simulink model "FlatEarth_MATLAB7"  (Simulink 8.1)
settings: Solver=ode45  StartTime=0.0  StopTime=Tstop  RelTol=1e-3
undefined symbols (not defined in the file): constant, deltaApertRAD, deltabhppert, deltaEpertRAD, deltaRpertRAD, sigbuilder_block, uIC, Xa, xIC
settings Model: Creator=andrisan  LastModifiedBy=Willdog  ExtModeAutoUpdateStatusClock=off
settings DataIOCC: SignalLoggingName=sigsOut
settings OptimizationCC: BooleanDataType=off  InitFltsAndDblsToZero=on
settings DebuggingCC: SaveWithParameterizedLinksMsg=none  SignalResolutionControl=TryResolveAllWithWarning  SolverPrmCheckMsg=none  MultiTaskDSMMsg=warning  MultiTaskCondExecSysMsg=none  StrictBusMsg=None
settings HardwareCC: TargetUnknown=on
settings RTWCC: IncludeERTFirstTime=on
settings GRTTargetCC: TargetFcnLib=ansi_tfl_tmw.mat

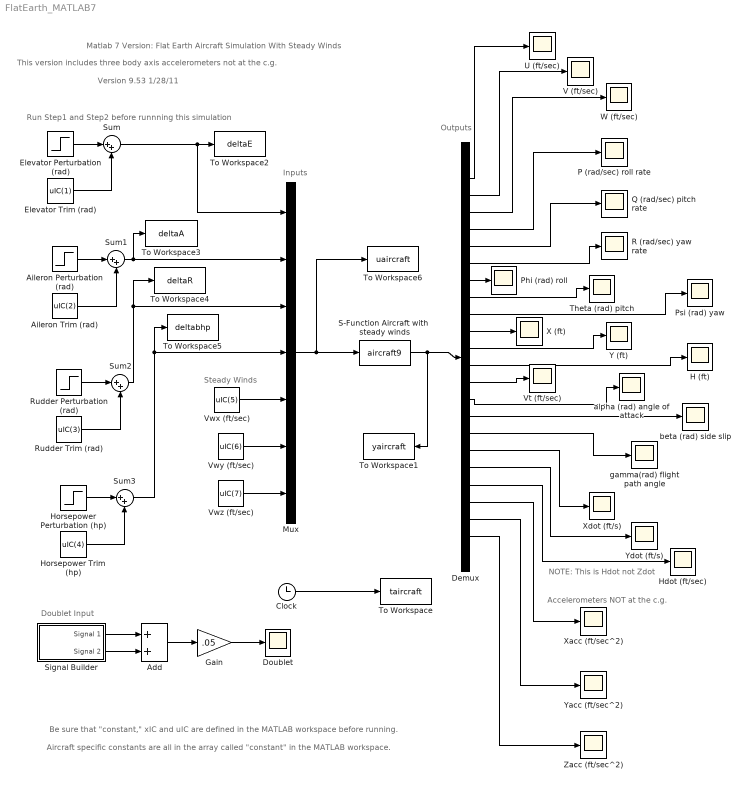
== system FlatEarth_MATLAB7 ==
  note: Matlab 7 Version: Flat Earth Aircraft Simulation With Steady Winds
  note: Version 9.53 1/28/11
  note: Be sure that "constant," xIC and uIC are defined in the MATLAB workspace before running.
  note: Aircraft specific constants are all in the array called "constant" in the MATLAB workspace.
  note: Steady Winds
  note: Inputs
  note: Outputs
  note: Run Step1 and Step2 before runnning this simulation
  note: This version includes three body axis accelerometers not at the c.g.
  note: Accelerometers NOT at the c.g.
  note: NOTE: This is Hdot not Zdot
  note: Doublet Input
  Add : Sum
  Aileron Perturbation (rad) : Step  After=deltaApertRAD  SampleTime=0
  Aileron Trim (rad) : Constant  Value=uIC(2)
  Clock : Clock
  Demux : Demux  Outputs=22
  Doublet : Scope
      settings: SaveName=ScopeData22
  Elevator Perturbation (rad) : Step  After=deltaEpertRAD  SampleTime=0
  Elevator Trim (rad) : Constant  Value=uIC(1)
  Gain : Gain  Gain=.05
  H (ft) : Scope
      settings: TimeRange=50  SaveName=ScopeData11
  Hdot (ft/sec) : Scope
      settings: SaveName=ScopeData18
  Horsepower Perturbation (hp) : Step  After=deltabhppert  SampleTime=0
  Horsepower Trim (hp) : Constant  Value=uIC(4)
  Mux : Mux  Inputs=7
  P (rad/sec) roll rate : Scope
      settings: SaveName=ScopeData3
  Phi (rad) roll : Scope
      settings: SaveName=ScopeData6
  Psi (rad) yaw : Scope
      settings: SaveName=ScopeData8
  Q (rad/sec) pitch rate : Scope
      settings: SaveName=ScopeData4
  R (rad/sec) yaw rate : Scope
      settings: SaveName=ScopeData5
  Rudder Perturbation (rad) : Step  After=deltaRpertRAD  SampleTime=0
  Rudder Trim (rad) : Constant  Value=uIC(3)
  S-Function Aircraft with  steady winds : S-Function  FunctionName=aircraft9  Parameters=constant,xIC,Xa  EnableBusSupport=off
  Signal Builder : Subsystem  Tag=STV Subsys  LoadFcn=sigbuilder_block('load');  StartFcn=sigbuilder_block('start');  StopFcn=sigbuilder_block('stop');  ClipboardFcn=sigbuilder_block('clipboard');  mask(Sigbuilder block){}
      mask help: Sigbuilder GUI
      mask init:
      | if ~strcmp(get_param(bdroot(gcbh),'SimulationStatus'),'stopped') tuvar = sigbuilder_block('maskInit'); end
      settings: CopyFcn=sigbuilder_block('copy');  DeleteFcn=sigbuilder_block('delete');  ModelCloseFcn=sigbuilder_block('modelClose');  PreSaveFcn=sigbuilder_block('preSave');  PauseFcn=sigbuilder_block('pause')  ContinueFcn=sigbuilder_block('continue')  NameChangeFcn=sigbuilder_block('namechange');  OpenFcn=sigbuilder_block('open',[437.6 199.2 550.4 400 ]);  CloseFcn=sigbuilder_block('close');
      mask Display: plot(0,0,100,100,[10,10,40,40,10],[80,20,20,80,80],[40,10],[50,50], [40,27,10],[65,72,56],[40,25,25,10],[28,28,43,43]);
  Sum{,1..3} (4 alike) : Sum  Inputs=|++  SaturateOnIntegerOverflow=on  InputSameDT=on  OutDataTypeStr=Inherit: Same as first input
  Theta (rad) pitch : Scope
      settings: SaveName=ScopeData7
  To Workspace : ToWorkspace  VariableName=taircraft  SampleTime=-1
  To Workspace1 : ToWorkspace  VariableName=yaircraft  SampleTime=-1
  To Workspace2 : ToWorkspace  VariableName=deltaE  SampleTime=-1
  To Workspace3 : ToWorkspace  VariableName=deltaA  SampleTime=-1
  To Workspace4 : ToWorkspace  VariableName=deltaR  SampleTime=-1
  To Workspace5 : ToWorkspace  VariableName=deltabhp  SampleTime=-1
  To Workspace6 : ToWorkspace  VariableName=uaircraft  SampleTime=-1
  U (ft/sec) : Scope
  V (ft/sec) : Scope
  Vt (ft/sec) : Scope
      settings: TimeRange=50  YMin=99.319  YMax=99.324  SaveName=ScopeData12
  Vwx (ft/sec) : Constant  Value=uIC(5)
  Vwy (ft/sec) : Constant  Value=uIC(6)
  Vwz (ft/sec) : Constant  Value=uIC(7)
  W (ft/sec) : Scope
      settings: YMin=0  YMax=14  SaveName=ScopeData2
  X (ft) : Scope
      settings: SaveName=ScopeData9
  Xacc (ft/sec^2) : Scope
      settings: SaveName=ScopeData19
  Xdot (ft/s) : Scope
      settings: SaveName=ScopeData16
  Y (ft) : Scope
      settings: SaveName=ScopeData10
  Yacc (ft/sec^2) : Scope
      settings: SaveName=ScopeData20
  Ydot (ft/s) : Scope
      settings: SaveName=ScopeData17
  Zacc (ft/sec^2) : Scope
      settings: SaveName=ScopeData21
  alpha (rad) angle of attack : Scope
      settings: SaveName=ScopeData13
  beta (rad) side slip : Scope
      settings: SaveName=ScopeData14
  gamma(rad) flight path angle : Scope
      settings: SaveName=ScopeData15
  wires:
  Demux/1 -> U (ft/sec)/1
  Demux/2 -> V (ft/sec)/1
  Demux/3 -> W (ft/sec)/1
  Demux/4 -> P (rad/sec) roll rate/1
  Demux/5 -> Q (rad/sec) pitch rate/1
  Demux/6 -> R (rad/sec) yaw rate/1
  Demux/7 -> Phi (rad) roll/1
  Demux/8 -> Theta (rad) pitch/1
  Demux/9 -> Psi (rad) yaw/1
  Demux/10 -> X (ft)/1
  Demux/11 -> Y (ft)/1
  Demux/12 -> H (ft)/1
  Demux/13 -> Vt (ft/sec)/1
  Demux/14 -> alpha (rad) angle of attack/1
  Demux/15 -> beta (rad) side slip/1
  Demux/16 -> gamma(rad) flight path angle/1
  Demux/17 -> Xdot (ft/s)/1
  Demux/18 -> Ydot (ft/s)/1
  Demux/19 -> Hdot (ft/sec)/1
  Clock/1 -> To Workspace/1
  S-Function Aircraft with  steady winds/1 -> Demux/1, To Workspace1/1
  Elevator Perturbation (rad)/1 -> Sum/1
  Elevator Trim (rad)/1 -> Sum/2
  Aileron Perturbation (rad)/1 -> Sum1/1
  Aileron Trim (rad)/1 -> Sum1/2
  Rudder Perturbation (rad)/1 -> Sum2/1
  Rudder Trim (rad)/1 -> Sum2/2
  Horsepower Perturbation (hp)/1 -> Sum3/1
  Horsepower Trim (hp)/1 -> Sum3/2
  Sum/1 -> Mux/1, To Workspace2/1
  Sum1/1 -> Mux/2, To Workspace3/1
  Sum2/1 -> Mux/3, To Workspace4/1
  Sum3/1 -> Mux/4, To Workspace5/1
  Vwx (ft/sec)/1 -> Mux/5
  Vwy (ft/sec)/1 -> Mux/6
  Vwz (ft/sec)/1 -> Mux/7
  Mux/1 -> S-Function Aircraft with  steady winds/1, To Workspace6/1
  Demux/20 -> Xacc (ft/sec^2)/1
  Demux/21 -> Yacc (ft/sec^2)/1
  Demux/22 -> Zacc (ft/sec^2)/1
  Signal Builder/1(Signal 1) -> Add/1
  Signal Builder/2(Signal 2) -> Add/2
  Add/1 -> Gain/1
  Gain/1 -> Doublet/1

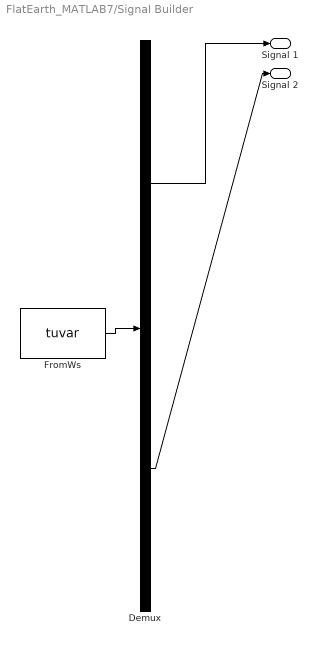
== system FlatEarth_MATLAB7/Signal Builder ==
  Demux : Demux  Tag=STV Demux  Outputs=2
  FromWs : FromWorkspace  Tag=STV FromWs  VariableName=tuvar  SampleTime=0  SigBuilderData=DataTag0  VnvData=DataTag1
      SigBuilderData=|
      | common.afterFinalStr = 'Extrapolate'
      | common.sampleTime = 0
      | dataSet.timeRange = [0 10]
      | dataSet.name = 'Group 1'
      | sbobj.Groups.Name = 'Group 1'
      | sbobj.Groups.Signals(1).Name = 'Signal 1'
      | sbobj.Groups.Signals(1).XData = [0 1 1 2 2 10]
      | sbobj.Groups.Signals(1).YData = [0 0 1 1 0 0]
      | sbobj.Groups.Signals(2).Name = 'Signal 2'
      | sbobj.Groups.Signals(2).XData = [0 2 2 3 3 10]
      | sbobj.Groups.Signals(2).YData = [0 0 -1 -1 0 0]
  Signal 1 : Outport  Tag=STV Outport
  Signal 2 : Outport  Tag=STV Outport  Port=2
  wires:
  Demux/1 -> Signal 1/1
  FromWs/1 -> Demux/1
  Demux/2 -> Signal 2/1
